simulink model "Four_phase_synch_buck"  (R2025a)
settings: Solver=VariableStepAuto  StartTime=0.0  StopTime=10  RelTol=1e-3
libraries: spsMosfetLib x8, spsGroundLib x6, spsSeriesRLCBranchLib x6, spsCurrentMeasurementLib x5, spsDCVoltageSourceLib x1, spsVoltageMeasurementLib x1, sps_lib x1
settings Model: Creator=HP  LastModifiedBy=HP

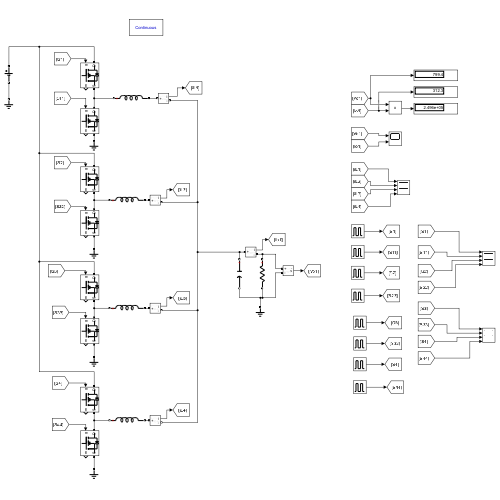
[thumbnail: Simulink's stored preview of the top-level diagram]
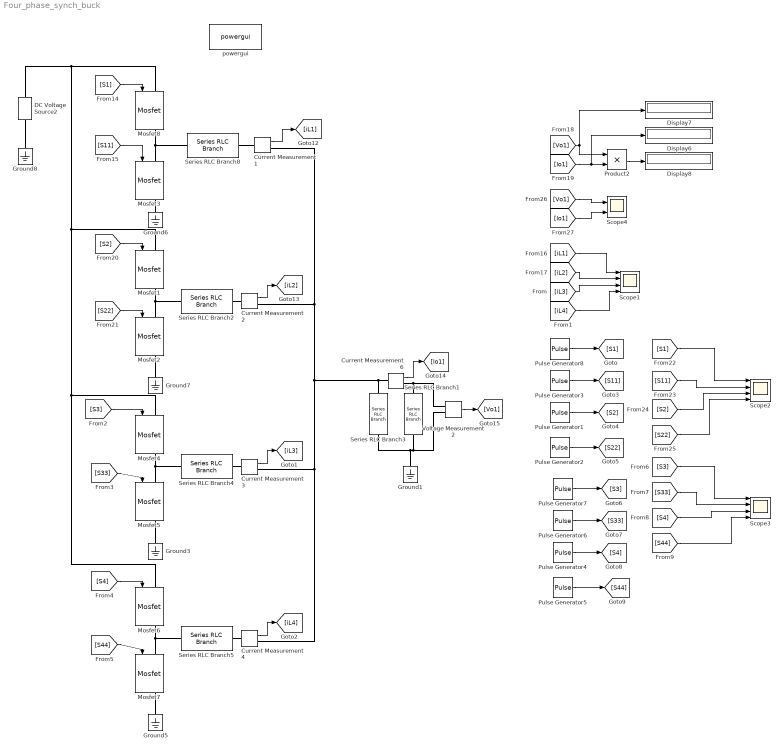
== system Four_phase_synch_buck ==
  Current Measurement{1..4,6} (5 alike) : spsCurrentMeasurementLib/Current Measurement  PhasorSimulation=off  OutputType=Complex  PSBequivalent=0
  DC Voltage Source2 : spsDCVoltageSourceLib/DC Voltage Source  Amplitude=1500  Measurements=None
  Display6 : Display
  Display7 : Display
  Display8 : Display
  Ground{1,3,5..8} (6 alike) : spsGroundLib/Ground  LConnTagsString=a
  Mosfet1 : spsMosfetLib/Mosfet  Ron=000.001  Lon=0  Rd=0.001  Vfd=0  IC=0  Rs=1e5  Cs=inf  Measurements=on
  Mosfet{2..3,5,7..8} (5 alike) : spsMosfetLib/Mosfet  Ron=0.001  Lon=0  Rd=0.001  Vfd=0  IC=0  Rs=1e5  Cs=inf  Measurements=on
  Mosfet4 : spsMosfetLib/Mosfet  Ron=000.001  Lon=0  Rd=0.001  Vfd=0  IC=0  Rs=1e5  Cs=inf  Measurements=on
  Mosfet6 : spsMosfetLib/Mosfet  Ron=000.001  Lon=0  Rd=0.001  Vfd=0  IC=0  Rs=1e5  Cs=inf  Measurements=on
  Product2 : Product
  Pulse Generator1 : DiscretePulseGenerator  PulseType=Time based  Period=1/35000  PulseWidth=53.3  PhaseDelay=7.442857143e-6
  Pulse Generator2 : DiscretePulseGenerator  PulseType=Time based  Period=1/35000  PulseWidth=44.6  PhaseDelay=22.97142857e-6
  Pulse Generator3 : DiscretePulseGenerator  PulseType=Time based  Period=1/35000  PulseWidth=44.6  PhaseDelay=15.82857143e-6
  Pulse Generator4 : DiscretePulseGenerator  PulseType=Time based  Period=1/35000  PulseWidth=53.3  PhaseDelay=21.7285714e-6
  Pulse Generator5 : DiscretePulseGenerator  PulseType=Time based  Period=1/35000  PulseWidth=44.6  PhaseDelay=8.38571429e-6
  Pulse Generator6 : DiscretePulseGenerator  PulseType=Time based  Period=1/35000  PulseWidth=44.6  PhaseDelay=1.54285714e-6
  Pulse Generator7 : DiscretePulseGenerator  PulseType=Time based  Period=1/35000  PulseWidth=53.3  PhaseDelay=14.58571429e-6
  Pulse Generator8 : DiscretePulseGenerator  PulseType=Time based  Period=1/35000  PulseWidth=53.3  PhaseDelay=300e-9
  Scope1 : Scope  NumInputPorts=4
      settings: ActiveDisplayString=4  Title=iL4  ActiveDisplayYMinimum=24.107232250576352  ActiveDisplayYMaximum=79.9270452727493
  Scope2 : Scope  NumInputPorts=4
      settings: ActiveDisplayString=4  Title=S22  ActiveDisplayYMinimum=-0.11718749999999997  ActiveDisplayYMaximum=1.1328125
  Scope3 : Scope  NumInputPorts=4
      settings: ActiveDisplayString=4  Title=S44  ActiveDisplayYMinimum=-0.12499999999999997  ActiveDisplayYMaximum=1.125  DataLoggingVariableName=ScopeData2
  Scope4 : Scope  NumInputPorts=2
      settings: ActiveDisplayYMinimum=-118.3454736321592  ActiveDisplayYMaximum=1066.6449481810444  DataLoggingVariableName=ScopeData4
  Series RLC Branch1 : spsSeriesRLCBranchLib/Series RLC Branch  LConnTagsString=__new0  RConnTagsString=__new0  BranchType=R  Resistance=2.56  Inductance=68e-6  SetiL0=off  InitialCurrent=0  Capacitance=55e-6  Setx0=off  InitialVoltage=0  Measurements=None
  Series RLC Branch{2,4..5,8} (4 alike) : spsSeriesRLCBranchLib/Series RLC Branch  LConnTagsString=__new0  RConnTagsString=__new0  BranchType=L  Resistance=1  Inductance=350e-6  SetiL0=off  InitialCurrent=0  Capacitance=1e-6  Setx0=off  InitialVoltage=0  Measurements=None
  Series RLC Branch3 : spsSeriesRLCBranchLib/Series RLC Branch  LConnTagsString=__new0  RConnTagsString=__new0  BranchType=C  Resistance=1  Inductance=68e-6  SetiL0=off  InitialCurrent=0  Capacitance=15e-6  Setx0=off  InitialVoltage=0  Measurements=None
  Voltage Measurement2 : spsVoltageMeasurementLib/Voltage Measurement  PhasorSimulation=off  OutputType=Complex  PSBequivalent=0
  powergui : sps_lib/powergui  Priority=1  SimulationMode=Continuous  SampleTime=2e-8  frequency=60  Iterations=50  frequencyindice=0  Pbase=100e6  ErrMax=1e-4  UnitsV=kV  UnitsW=MW  buscounter=0  FunctionMessages=off  echomessages=off  EnableUseOfTLC=off  CurrentSourceSwitches=off  DisableSnubberDevices=off  DisableRonSwitches=off  DisableVfSwitches=off  DisplayEquations=off  AutomaticDiscreteSolvers=off  SolverType=Tustin/Backward Euler (TBE)  Interpol=off  ExternalGateDelay=off  methode=off  Ts=100  x0status=blocks  SPID=on  SwTol=0  HookPort=off  NonlinearTolerance=1e-4  nMaxIteration=100  ContinueOnMaxIteration=off  RestoreLinks=warning  ResistiveCurrentMeasurement=off  Frange=[0:2:500]  Ylog=off  Xlog=on  ShowGrid=off  save=off  variable=ZData  structure=0  ZoomFFT=off  StartTime=0.0  cycles=1  DisplayStyle=1  fundamental=60  FreqAxis=off  MaxFrequency=1000  frequencyindicesteady=1  RmsSteady=1  display=off
  wires:
  [Io1] -> Scope4/2
  [Io1] -> Display6/1, Product2/2
  Current Measurement6/1 -> [Io1]
  [Vo1] -> Scope4/1
  Pulse Generator3/1 -> [S11]
  [S2] -> Mosfet1/1
  [Vo1] -> Display7/1, Product2/1
  [iL1] -> Scope1/1
  Pulse Generator2/1 -> [S22]
  Pulse Generator8/1 -> [S1]
  [S22] -> Mosfet2/1
  Product2/1 -> Display8/1
  [S11] -> Mosfet3/1
  Voltage Measurement2/1 -> [Vo1]
  [S1] -> Mosfet8/1
  Current Measurement2/1 -> [iL2]
  Pulse Generator1/1 -> [S2]
  Current Measurement1/1 -> [iL1]
  [iL2] -> Scope1/2
  [iL3] -> Scope1/3
  [iL4] -> Scope1/4
  Current Measurement3/1 -> [iL3]
  [S33] -> Mosfet5/1
  [S3] -> Mosfet4/1
  Current Measurement4/1 -> [iL4]
  [S44] -> Mosfet7/1
  [S4] -> Mosfet6/1
  Pulse Generator4/1 -> [S4]
  Pulse Generator7/1 -> [S3]
  Pulse Generator5/1 -> [S44]
  Pulse Generator6/1 -> [S33]
  [S1] -> Scope2/1
  [S11] -> Scope2/2
  [S2] -> Scope2/3
  [S22] -> Scope2/4
  [S3] -> Scope3/1
  [S33] -> Scope3/2
  [S4] -> Scope3/3
  [S44] -> Scope3/4
  connections:
  Current Measurement6/LConn1 -- Series RLC Branch3/LConn1 -- Current Measurement4/RConn1 -- Current Measurement3/RConn1 -- Current Measurement1/RConn1 -- Current Measurement2/RConn1
  Mosfet2/LConn1 -- Mosfet1/RConn1 -- Series RLC Branch2/LConn1
  Series RLC Branch1/RConn1 -- Series RLC Branch3/RConn1 -- Ground1/LConn1 -- Voltage Measurement2/LConn2
  Mosfet8/RConn1 -- Mosfet3/LConn1 -- Series RLC Branch8/LConn1
  Mosfet1/LConn1 -- Mosfet4/LConn1 -- Mosfet6/LConn1 -- Mosfet8/LConn1 -- DC Voltage Source2/RConn1
  Voltage Measurement2/LConn1 -- Current Measurement6/RConn1 -- Series RLC Branch1/LConn1
  DC Voltage Source2/LConn1 -- Ground8/LConn1
  Ground7/LConn1 -- Mosfet2/RConn1
  Ground6/LConn1 -- Mosfet3/RConn1
  Current Measurement1/LConn1 -- Series RLC Branch8/RConn1
  Current Measurement2/LConn1 -- Series RLC Branch2/RConn1
  Mosfet5/LConn1 -- Series RLC Branch4/LConn1 -- Mosfet4/RConn1
  Current Measurement3/LConn1 -- Series RLC Branch4/RConn1
  Ground3/LConn1 -- Mosfet5/RConn1
  Mosfet7/LConn1 -- Series RLC Branch5/LConn1 -- Mosfet6/RConn1
  Current Measurement4/LConn1 -- Series RLC Branch5/RConn1
  Ground5/LConn1 -- Mosfet7/RConn1
